simulink library "calc_radius_of_curvature"  (R2020a)
settings: Solver=VariableStepAuto  StartTime=0.0  StopTime=10.0  RelTol=1e-3
settings Model: Creator=Ayaz  LastModifiedBy=Ayaz

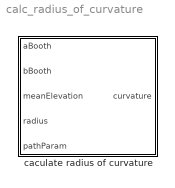
== system calc_radius_of_curvature ==
  caculate radius of curvature : Subsystem

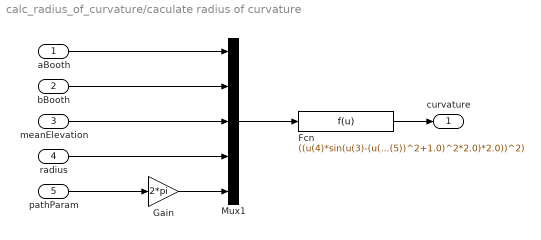
== system calc_radius_of_curvature/caculate radius of curvature ==
  aBooth : Inport
  bBooth : Inport  Port=2
  meanElevation : Inport  Port=3
  radius : Inport  Port=4
  pathParam : Inport  Port=5
  Fcn : Fcn  Expr=((u(4)*sin(u(3)-(u(1)^2*1.0/u(2)^2*cos(u(5))*sin(u(5)))/(u(1)^2*1.0/u(2)^2*cos(u(5))^2+1.0))*sin((u(1)*sin(u(5)))/(u(1)^2*1.0/u(2)^2*cos(u(5))^2+1.0))*((u(1)^2*1.0/u(2)^2*cos(u(5))^2)/(u(1)^2*1.0/u(2)^2*cos(u(5))^2+1.0)-(u(1)^2*1.0/u(2)^2*sin(u(5))^2)/(u(1)^2*1.0/u(2)^2*cos(u(5))^2+1.0)+u(1)^4*1.0/u(2)^4*cos(u(5))^2*sin(u(5))^2*1.0/(u(1)^2*1.0/u(2)^2*cos(u(5))^2+1.0)^2*2.0)+u(4)*cos(u(3)-(u(1)^2*1.0/u(2)^2*cos(u(5))*sin(u(5)))/(u(1)^2*1.0/u(2)^2*cos(u(5))^2+1.0))*cos((u(1)*sin(u(5)))/(u(1)^2*1.0/u(2)^2*cos(u(5))^2+1.0))*((u(1)*cos(u(5)))/(u(1)^2*1.0/u(2)^2*cos(u(5))^2+1.0)+u(1)^3*1.0/u(2)^2*cos(u(5))*sin(u(5))^2*1.0/(u(1)^2*1.0/u(2)^2*cos(u(5))^2+1.0)^2*2.0))^2+(u(4)*sin(u(3)-(u(1)^2*1.0/u(2)^2*cos(u(5))*sin(u(5)))/(u(1)^2*1.0/u(2)^2*cos(u(5))^2+1.0))*cos((u(1)*sin(u(5)))/(u(1)^2*1.0/u(2)^2*cos(u(5))^2+1.0))*((u(1)^2*1.0/u(2)^2*cos(u(5))^2)/(u(1)^2*1.0/u(2)^2*cos(u(5))^2+1.0)-(u(1)^2*1.0/u(2)^2*sin(u(5))^2)/(u(1)^2*1.0/u(2)^2*cos(u(5))^2+1.0)+u(1)^4*1.0/u(2)^4*cos(u(5))^2*sin(u(5))^2*1.0/(u(1)^2*1.0/u(2)^2*cos(u(5))^2+1.0)^2*2.0)-u(4)*cos(u(3)-(u(1)^2*1.0/u(2)^2*cos(u(5))*sin(u(5)))/(u(1)^2*1.0/u(2)^2*cos(u(5))^2+1.0))*sin((u(1)*sin(u(5)))/(u(1)^2*1.0/u(2)^2*cos(u(5))^2+1.0))*((u(1)*cos(u(5)))/(u(1)^2*1.0/u(2)^2*cos(u(5))^2+1.0)+u(1)^3*1.0/u(2)^2*cos(u(5))*sin(u(5))^2*1.0/(u(1)^2*1.0/u(2)^2*cos(u(5))^2+1.0)^2*2.0))^2+u(4)^2*cos(u(3)-(u(1)^2*1.0/u(2)^2*cos(u(5))*sin(u(5)))/(u(1)^2*1.0/u(2)^2*cos(u(5))^2+1.0))^2*((u(1)^2*1.0/u(2)^2*cos(u(5))^2)/(u(1)^2*1.0/u(2)^2*cos(u(5))^2+1.0)-(u(1)^2*1.0/u(2)^2*sin(u(5))^2)/(u(1)^2*1.0/u(2)^2*cos(u(5))^2+1.0)+u(1)^4*1.0/u(2)^4*cos(u(5))^2*sin(u(5))^2*1.0/(u(1)^2*1.0/u(2)^2*cos(u(5))^2+1.0)^2*2.0)^2)^(3.0/2.0)*1.0/sqrt(((u(4)*sin(u(3)-(u(1)^2*1.0/u(2)^2*cos(u(5))*sin(u(5)))/(u(1)^2*1.0/u(2)^2*cos(u(5))^2+1.0))*cos((u(1)*sin(u(5)))/(u(1)^2*1.0/u(2)^2*cos(u(5))^2+1.0))*((u(1)^2*1.0/u(2)^2*cos(u(5))^2)/(u(1)^2*1.0/u(2)^2*cos(u(5))^2+1.0)-(u(1)^2*1.0/u(2)^2*sin(u(5))^2)/(u(1)^2*1.0/u(2)^2*cos(u(5))^2+1.0)+u(1)^4*1.0/u(2)^4*cos(u(5))^2*sin(u(5))^2*1.0/(u(1)^2*1.0/u(2)^2*cos(u(5))^2+1.0)^2*2.0)-u(4)*cos(u(3)-(u(1)^2*1.0/u(2)^2*cos(u(5))*sin(u(5)))/(u(1)^2*1.0/u(2)^2*cos(u(5))^2+1.0))*sin((u(1)*sin(u(5)))/(u(1)^2*1.0/u(2)^2*cos(u(5))^2+1.0))*((u(1)*cos(u(5)))/(u(1)^2*1.0/u(2)^2*cos(u(5))^2+1.0)+u(1)^3*1.0/u(2)^2*cos(u(5))*sin(u(5))^2*1.0/(u(1)^2*1.0/u(2)^2*cos(u(5))^2+1.0)^2*2.0))*(u(4)*cos(u(3)-(u(1)^2*1.0/u(2)^2*cos(u(5))*sin(u(5)))/(u(1)^2*1.0/u(2)^2*cos(u(5))^2+1.0))*(u(1)^6*1.0/u(2)^6*cos(u(5))^3*sin(u(5))^3*1.0/(u(1)^2*1.0/u(2)^2*cos(u(5))^2+1.0)^3*8.0-(u(1)^2*1.0/u(2)^2*cos(u(5))*sin(u(5))*4.0)/(u(1)^2*1.0/u(2)^2*cos(u(5))^2+1.0)-u(1)^4*1.0/u(2)^4*cos(u(5))*sin(u(5))^3*1.0/(u(1)^2*1.0/u(2)^2*cos(u(5))^2+1.0)^2*6.0+u(1)^4*1.0/u(2)^4*cos(u(5))^3*sin(u(5))*1.0/(u(1)^2*1.0/u(2)^2*cos(u(5))^2+1.0)^2*6.0)+u(4)*sin(u(3)-(u(1)^2*1.0/u(2)^2*cos(u(5))*sin(u(5)))/(u(1)^2*1.0/u(2)^2*cos(u(5))^2+1.0))*((u(1)^2*1.0/u(2)^2*cos(u(5))^2)/(u(1)^2*1.0/u(2)^2*cos(u(5))^2+1.0)-(u(1)^2*1.0/u(2)^2*sin(u(5))^2)/(u(1)^2*1.0/u(2)^2*cos(u(5))^2+1.0)+u(1)^4*1.0/u(2)^4*cos(u(5))^2*sin(u(5))^2*1.0/(u(1)^2*1.0/u(2)^2*cos(u(5))^2+1.0)^2*2.0)^2)+u(4)*cos(u(3)-(u(1)^2*1.0/u(2)^2*cos(u(5))*sin(u(5)))/(u(1)^2*1.0/u(2)^2*cos(u(5))^2+1.0))*((u(1)^2*1.0/u(2)^2*cos(u(5))^2)/(u(1)^2*1.0/u(2)^2*cos(u(5))^2+1.0)-(u(1)^2*1.0/u(2)^2*sin(u(5))^2)/(u(1)^2*1.0/u(2)^2*cos(u(5))^2+1.0)+u(1)^4*1.0/u(2)^4*cos(u(5))^2*sin(u(5))^2*1.0/(u(1)^2*1.0/u(2)^2*cos(u(5))^2+1.0)^2*2.0)*(u(4)*cos(u(3)-(u(1)^2*1.0/u(2)^2*cos(u(5))*sin(u(5)))/(u(1)^2*1.0/u(2)^2*cos(u(5))^2+1.0))*cos((u(1)*sin(u(5)))/(u(1)^2*1.0/u(2)^2*cos(u(5))^2+1.0))*((u(1)^2*1.0/u(2)^2*cos(u(5))^2)/(u(1)^2*1.0/u(2)^2*cos(u(5))^2+1.0)-(u(1)^2*1.0/u(2)^2*sin(u(5))^2)/(u(1)^2*1.0/u(2)^2*cos(u(5))^2+1.0)+u(1)^4*1.0/u(2)^4*cos(u(5))^2*sin(u(5))^2*1.0/(u(1)^2*1.0/u(2)^2*cos(u(5))^2+1.0)^2*2.0)^2-u(4)*cos(u(3)-(u(1)^2*1.0/u(2)^2*cos(u(5))*sin(u(5)))/(u(1)^2*1.0/u(2)^2*cos(u(5))^2+1.0))*sin((u(1)*sin(u(5)))/(u(1)^2*1.0/u(2)^2*cos(u(5))^2+1.0))*((u(1)*sin(u(5)))/(u(1)^2*1.0/u(2)^2*cos(u(5))^2+1.0)+u(1)^3*1.0/u(2)^2*sin(u(5))^3*1.0/(u(1)^2*1.0/u(2)^2*cos(u(5))^2+1.0)^2*2.0-u(1)^5*1.0/u(2)^4*cos(u(5))^2*sin(u(5))^3*1.0/(u(1)^2*1.0/u(2)^2*cos(u(5))^2+1.0)^3*8.0-u(1)^3*1.0/u(2)^2*cos(u(5))^2*sin(u(5))*1.0/(u(1)^2*1.0/u(2)^2*cos(u(5))^2+1.0)^2*6.0)+u(4)*cos(u(3)-(u(1)^2*1.0/u(2)^2*cos(u(5))*sin(u(5)))/(u(1)^2*1.0/u(2)^2*cos(u(5))^2+1.0))*cos((u(1)*sin(u(5)))/(u(1)^2*1.0/u(2)^2*cos(u(5))^2+1.0))*((u(1)*cos(u(5)))/(u(1)^2*1.0/u(2)^2*cos(u(5))^2+1.0)+u(1)^3*1.0/u(2)^2*cos(u(5))*sin(u(5))^2*1.0/(u(1)^2*1.0/u(2)^2*cos(u(5))^2+1.0)^2*2.0)^2-u(4)*sin(u(3)-(u(1)^2*1.0/u(2)^2*cos(u(5))*sin(u(5)))/(u(1)^2*1.0/u(2)^2*cos(u(5))^2+1.0))*cos((u(1)*sin(u(5)))/(u(1)^2*1.0/u(2)^2*cos(u(5))^2+1.0))*(u(1)^6*1.0/u(2)^6*cos(u(5))^3*sin(u(5))^3*1.0/(u(1)^2*1.0/u(2)^2*cos(u(5))^2+1.0)^3*8.0-(u(1)^2*1.0/u(2)^2*cos(u(5))*sin(u(5))*4.0)/(u(1)^2*1.0/u(2)^2*cos(u(5))^2+1.0)-u(1)^4*1.0/u(2)^4*cos(u(5))*sin(u(5))^3*1.0/(u(1)^2*1.0/u(2)^2*cos(u(5))^2+1.0)^2*6.0+u(1)^4*1.0/u(2)^4*cos(u(5))^3*sin(u(5))*1.0/(u(1)^2*1.0/u(2)^2*cos(u(5))^2+1.0)^2*6.0)+u(4)*sin(u(3)-(u(1)^2*1.0/u(2)^2*cos(u(5))*sin(u(5)))/(u(1)^2*1.0/u(2)^2*cos(u(5))^2+1.0))*sin((u(1)*sin(u(5)))/(u(1)^2*1.0/u(2)^2*cos(u(5))^2+1.0))*((u(1)*cos(u(5)))/(u(1)^2*1.0/u(2)^2*cos(u(5))^2+1.0)+u(1)^3*1.0/u(2)^2*cos(u(5))*sin(u(5))^2*1.0/(u(1)^2*1.0/u(2)^2*cos(u(5))^2+1.0)^2*2.0)*((u(1)^2*1.0/u(2)^2*cos(u(5))^2)/(u(1)^2*1.0/u(2)^2*cos(u(5))^2+1.0)-(u(1)^2*1.0/u(2)^2*sin(u(5))^2)/(u(1)^2*1.0/u(2)^2*cos(u(5))^2+1.0)+u(1)^4*1.0/u(2)^4*cos(u(5))^2*sin(u(5))^2*1.0/(u(1)^2*1.0/u(2)^2*cos(u(5))^2+1.0)^2*2.0)*2.0))^2+((u(4)*sin(u(3)-(u(1)^2*1.0/u(2)^2*cos(u(5))*sin(u(5)))/(u(1)^2*1.0/u(2)^2*cos(u(5))^2+1.0))*sin((u(1)*sin(u(5)))/(u(1)^2*1.0/u(2)^2*cos(u(5))^2+1.0))*((u(1)^2*1.0/u(2)^2*cos(u(5))^2)/(u(1)^2*1.0/u(2)^2*cos(u(5))^2+1.0)-(u(1)^2*1.0/u(2)^2*sin(u(5))^2)/(u(1)^2*1.0/u(2)^2*cos(u(5))^2+1.0)+u(1)^4*1.0/u(2)^4*cos(u(5))^2*sin(u(5))^2*1.0/(u(1)^2*1.0/u(2)^2*cos(u(5))^2+1.0)^2*2.0)+u(4)*cos(u(3)-(u(1)^2*1.0/u(2)^2*cos(u(5))*sin(u(5)))/(u(1)^2*1.0/u(2)^2*cos(u(5))^2+1.0))*cos((u(1)*sin(u(5)))/(u(1)^2*1.0/u(2)^2*cos(u(5))^2+1.0))*((u(1)*cos(u(5)))/(u(1)^2*1.0/u(2)^2*cos(u(5))^2+1.0)+u(1)^3*1.0/u(2)^2*cos(u(5))*sin(u(5))^2*1.0/(u(1)^2*1.0/u(2)^2*cos(u(5))^2+1.0)^2*2.0))*(u(4)*cos(u(3)-(u(1)^2*1.0/u(2)^2*cos(u(5))*sin(u(5)))/(u(1)^2*1.0/u(2)^2*cos(u(5))^2+1.0))*(u(1)^6*1.0/u(2)^6*cos(u(5))^3*sin(u(5))^3*1.0/(u(1)^2*1.0/u(2)^2*cos(u(5))^2+1.0)^3*8.0-(u(1)^2*1.0/u(2)^2*cos(u(5))*sin(u(5))*4.0)/(u(1)^2*1.0/u(2)^2*cos(u(5))^2+1.0)-u(1)^4*1.0/u(2)^4*cos(u(5))*sin(u(5))^3*1.0/(u(1)^2*1.0/u(2)^2*cos(u(5))^2+1.0)^2*6.0+u(1)^4*1.0/u(2)^4*cos(u(5))^3*sin(u(5))*1.0/(u(1)^2*1.0/u(2)^2*cos(u(5))^2+1.0)^2*6.0)+u(4)*sin(u(3)-(u(1)^2*1.0/u(2)^2*cos(u(5))*sin(u(5)))/(u(1)^2*1.0/u(2)^2*cos(u(5))^2+1.0))*((u(1)^2*1.0/u(2)^2*cos(u(5))^2)/(u(1)^2*1.0/u(2)^2*cos(u(5))^2+1.0)-(u(1)^2*1.0/u(2)^2*sin(u(5))^2)/(u(1)^2*1.0/u(2)^2*cos(u(5))^2+1.0)+u(1)^4*1.0/u(2)^4*cos(u(5))^2*sin(u(5))^2*1.0/(u(1)^2*1.0/u(2)^2*cos(u(5))^2+1.0)^2*2.0)^2)+u(4)*cos(u(3)-(u(1)^2*1.0/u(2)^2*cos(u(5))*sin(u(5)))/(u(1)^2*1.0/u(2)^2*cos(u(5))^2+1.0))*((u(1)^2*1.0/u(2)^2*cos(u(5))^2)/(u(1)^2*1.0/u(2)^2*cos(u(5))^2+1.0)-(u(1)^2*1.0/u(2)^2*sin(u(5))^2)/(u(1)^2*1.0/u(2)^2*cos(u(5))^2+1.0)+u(1)^4*1.0/u(2)^4*cos(u(5))^2*sin(u(5))^2*1.0/(u(1)^2*1.0/u(2)^2*cos(u(5))^2+1.0)^2*2.0)*(-u(4)*sin(u(3)-(u(1)^2*1.0/u(2)^2*cos(u(5))*sin(u(5)))/(u(1)^2*1.0/u(2)^2*cos(u(5))^2+1.0))*sin((u(1)*sin(u(5)))/(u(1)^2*1.0/u(2)^2*cos(u(5))^2+1.0))*(u(1)^6*1.0/u(2)^6*cos(u(5))^3*sin(u(5))^3*1.0/(u(1)^2*1.0/u(2)^2*cos(u(5))^2+1.0)^3*8.0-(u(1)^2*1.0/u(2)^2*cos(u(5))*sin(u(5))*4.0)/(u(1)^2*1.0/u(2)^2*cos(u(5))^2+1.0)-u(1)^4*1.0/u(2)^4*cos(u(5))*sin(u(5))^3*1.0/(u(1)^2*1.0/u(2)^2*cos(u(5))^2+1.0)^2*6.0+u(1)^4*1.0/u(2)^4*cos(u(5))^3*sin(u(5))*1.0/(u(1)^2*1.0/u(2)^2*cos(u(5))^2+1.0)^2*6.0)+u(4)*cos(u(3)-(u(1)^2*1.0/u(2)^2*cos(u(5))*sin(u(5)))/(u(1)^2*1.0/u(2)^2*cos(u(5))^2+1.0))*cos((u(1)*sin(u(5)))/(u(1)^2*1.0/u(2)^2*cos(u(5))^2+1.0))*((u(1)*sin(u(5)))/(u(1)^2*1.0/u(2)^2*cos(u(5))^2+1.0)+u(1)^3*1.0/u(2)^2*sin(u(5))^3*1.0/(u(1)^2*1.0/u(2)^2*cos(u(5))^2+1.0)^2*2.0-u(1)^5*1.0/u(2)^4*cos(u(5))^2*sin(u(5))^3*1.0/(u(1)^2*1.0/u(2)^2*cos(u(5))^2+1.0)^3*8.0-u(1)^3*1.0/u(2)^2*cos(u(5))^2*sin(u(5))*1.0/(u(1)^2*1.0/u(2)^2*cos(u(5))^2+1.0)^2*6.0)+u(4)*cos(u(3)-(u(1)^2*1.0/u(2)^2*cos(u(5))*sin(u(5)))/(u(1)^2*1.0/u(2)^2*cos(u(5))^2+1.0))*sin((u(1)*sin(u(5)))/(u(1)^2*1.0/u(2)^2*cos(u(5))^2+1.0))*((u(1)^2*1.0/u(2)^2*cos(u(5))^2)/(u(1)^2*1.0/u(2)^2*cos(u(5))^2+1.0)-(u(1)^2*1.0/u(2)^2*sin(u(5))^2)/(u(1)^2*1.0/u(2)^2*cos(u(5))^2+1.0)+u(1)^4*1.0/u(2)^4*cos(u(5))^2*sin(u(5))^2*1.0/(u(1)^2*1.0/u(2)^2*cos(u(5))^2+1.0)^2*2.0)^2+u(4)*cos(u(3)-(u(1)^2*1.0/u(2)^2*cos(u(5))*sin(u(5)))/(u(1)^2*1.0/u(2)^2*cos(u(5))^2+1.0))*sin((u(1)*sin(u(5)))/(u(1)^2*1.0/u(2)^2*cos(u(5))^2+1.0))*((u(1)*cos(u(5)))/(u(1)^2*1.0/u(2)^2*cos(u(5))^2+1.0)+u(1)^3*1.0/u(2)^2*cos(u(5))*sin(u(5))^2*1.0/(u(1)^2*1.0/u(2)^2*cos(u(5))^2+1.0)^2*2.0)^2-u(4)*sin(u(3)-(u(1)^2*1.0/u(2)^2*cos(u(5))*sin(u(5)))/(u(1)^2*1.0/u(2)^2*cos(u(5))^2+1.0))*cos((u(1)*sin(u(5)))/(u(1)^2*1.0/u(2)^2*cos(u(5))^2+1.0))*((u(1)*cos(u(5)))/(u(1)^2*1.0/u(2)^2*cos(u(5))^2+1.0)+u(1)^3*1.0/u(2)^2*cos(u(5))*sin(u(5))^2*1.0/(u(1)^2*1.0/u(2)^2*cos(u(5))^2+1.0)^2*2.0)*((u(1)^2*1.0/u(2)^2*cos(u(5))^2)/(u(1)^2*1.0/u(2)^2*cos(u(5))^2+1.0)-(u(1)^2*1.0/u(2)^2*sin(u(5))^2)/(u(1)^2*1.0/u(2)^2*cos(u(5))^2+1.0)+u(1)^4*1.0/u(2)^4*cos(u(5))^2*sin(u(5))^2*1.0/(u(1)^2*1.0/u(2)^2*cos(u(5))^2+1.0)^2*2.0)*2.0))^2+((u(4)*sin(u(3)-(u(1)^2*1.0/u(2)^2*cos(u(5))*sin(u(5)))/(u(1)^2*1.0/u(2)^2*cos(u(5))^2+1.0))*sin((u(1)*sin(u(5)))/(u(1)^2*1.0/u(2)^2*cos(u(5))^2+1.0))*((u(1)^2*1.0/u(2)^2*cos(u(5))^2)/(u(1)^2*1.0/u(2)^2*cos(u(5))^2+1.0)-(u(1)^2*1.0/u(2)^2*sin(u(5))^2)/(u(1)^2*1.0/u(2)^2*cos(u(5))^2+1.0)+u(1)^4*1.0/u(2)^4*cos(u(5))^2*sin(u(5))^2*1.0/(u(1)^2*1.0/u(2)^2*cos(u(5))^2+1.0)^2*2.0)+u(4)*cos(u(3)-(u(1)^2*1.0/u(2)^2*cos(u(5))*sin(u(5)))/(u(1)^2*1.0/u(2)^2*cos(u(5))^2+1.0))*cos((u(1)*sin(u(5)))/(u(1)^2*1.0/u(2)^2*cos(u(5))^2+1.0))*((u(1)*cos(u(5)))/(u(1)^2*1.0/u(2)^2*cos(u(5))^2+1.0)+u(1)^3*1.0/u(2)^2*cos(u(5))*sin(u(5))^2*1.0/(u(1)^2*1.0/u(2)^2*cos(u(5))^2+1.0)^2*2.0))*(u(4)*cos(u(3)-(u(1)^2*1.0/u(2)^2*cos(u(5))*sin(u(5)))/(u(1)^2*1.0/u(2)^2*cos(u(5))^2+1.0))*cos((u(1)*sin(u(5)))/(u(1)^2*1.0/u(2)^2*cos(u(5))^2+1.0))*((u(1)^2*1.0/u(2)^2*cos(u(5))^2)/(u(1)^2*1.0/u(2)^2*cos(u(5))^2+1.0)-(u(1)^2*1.0/u(2)^2*sin(u(5))^2)/(u(1)^2*1.0/u(2)^2*cos(u(5))^2+1.0)+u(1)^4*1.0/u(2)^4*cos(u(5))^2*sin(u(5))^2*1.0/(u(1)^2*1.0/u(2)^2*cos(u(5))^2+1.0)^2*2.0)^2-u(4)*cos(u(3)-(u(1)^2*1.0/u(2)^2*cos(u(5))*sin(u(5)))/(u(1)^2*1.0/u(2)^2*cos(u(5))^2+1.0))*sin((u(1)*sin(u(5)))/(u(1)^2*1.0/u(2)^2*cos(u(5))^2+1.0))*((u(1)*sin(u(5)))/(u(1)^2*1.0/u(2)^2*cos(u(5))^2+1.0)+u(1)^3*1.0/u(2)^2*sin(u(5))^3*1.0/(u(1)^2*1.0/u(2)^2*cos(u(5))^2+1.0)^2*2.0-u(1)^5*1.0/u(2)^4*cos(u(5))^2*sin(u(5))^3*1.0/(u(1)^2*1.0/u(2)^2*cos(u(5))^2+1.0)^3*8.0-u(1)^3*1.0/u(2)^2*cos(u(5))^2*sin(u(5))*1.0/(u(1)^2*1.0/u(2)^2*cos(u(5))^2+1.0)^2*6.0)+u(4)*cos(u(3)-(u(1)^2*1.0/u(2)^2*cos(u(5))*sin(u(5)))/(u(1)^2*1.0/u(2)^2*cos(u(5))^2+1.0))*cos((u(1)*sin(u(5)))/(u(1)^2*1.0/u(2)^2*cos(u(5))^2+1.0))*((u(1)*cos(u(5)))/(u(1)^2*1.0/u(2)^2*cos(u(5))^2+1.0)+u(1)^3*1.0/u(2)^2*cos(u(5))*sin(u(5))^2*1.0/(u(1)^2*1.0/u(2)^2*cos(u(5))^2+1.0)^2*2.0)^2-u(4)*sin(u(3)-(u(1)^2*1.0/u(2)^2*cos(u(5))*sin(u(5)))/(u(1)^2*1.0/u(2)^2*cos(u(5))^2+1.0))*cos((u(1)*sin(u(5)))/(u(1)^2*1.0/u(2)^2*cos(u(5))^2+1.0))*(u(1)^6*1.0/u(2)^6*cos(u(5))^3*sin(u(5))^3*1.0/(u(1)^2*1.0/u(2)^2*cos(u(5))^2+1.0)^3*8.0-(u(1)^2*1.0/u(2)^2*cos(u(5))*sin(u(5))*4.0)/(u(1)^2*1.0/u(2)^2*cos(u(5))^2+1.0)-u(1)^4*1.0/u(2)^4*cos(u(5))*sin(u(5))^3*1.0/(u(1)^2*1.0/u(2)^2*cos(u(5))^2+1.0)^2*6.0+u(1)^4*1.0/u(2)^4*cos(u(5))^3*sin(u(5))*1.0/(u(1)^2*1.0/u(2)^2*cos(u(5))^2+1.0)^2*6.0)+u(4)*sin(u(3)-(u(1)^2*1.0/u(2)^2*cos(u(5))*sin(u(5)))/(u(1)^2*1.0/u(2)^2*cos(u(5))^2+1.0))*sin((u(1)*sin(u(5)))/(u(1)^2*1.0/u(2)^2*cos(u(5))^2+1.0))*((u(1)*cos(u(5)))/(u(1)^2*1.0/u(2)^2*cos(u(5))^2+1.0)+u(1)^3*1.0/u(2)^2*cos(u(5))*sin(u(5))^2*1.0/(u(1)^2*1.0/u(2)^2*cos(u(5))^2+1.0)^2*2.0)*((u(1)^2*1.0/u(2)^2*cos(u(5))^2)/(u(1)^2*1.0/u(2)^2*cos(u(5))^2+1.0)-(u(1)^2*1.0/u(2)^2*sin(u(5))^2)/(u(1)^2*1.0/u(2)^2*cos(u(5))^2+1.0)+u(1)^4*1.0/u(2)^4*cos(u(5))^2*sin(u(5))^2*1.0/(u(1)^2*1.0/u(2)^2*cos(u(5))^2+1.0)^2*2.0)*2.0)-(u(4)*sin(u(3)-(u(1)^2*1.0/u(2)^2*cos(u(5))*sin(u(5)))/(u(1)^2*1.0/u(2)^2*cos(u(5))^2+1.0))*cos((u(1)*sin(u(5)))/(u(1)^2*1.0/u(2)^2*cos(u(5))^2+1.0))*((u(1)^2*1.0/u(2)^2*cos(u(5))^2)/(u(1)^2*1.0/u(2)^2*cos(u(5))^2+1.0)-(u(1)^2*1.0/u(2)^2*sin(u(5))^2)/(u(1)^2*1.0/u(2)^2*cos(u(5))^2+1.0)+u(1)^4*1.0/u(2)^4*cos(u(5))^2*sin(u(5))^2*1.0/(u(1)^2*1.0/u(2)^2*cos(u(5))^2+1.0)^2*2.0)-u(4)*cos(u(3)-(u(1)^2*1.0/u(2)^2*cos(u(5))*sin(u(5)))/(u(1)^2*1.0/u(2)^2*cos(u(5))^2+1.0))*sin((u(1)*sin(u(5)))/(u(1)^2*1.0/u(2)^2*cos(u(5))^2+1.0))*((u(1)*cos(u(5)))/(u(1)^2*1.0/u(2)^2*cos(u(5))^2+1.0)+u(1)^3*1.0/u(2)^2*cos(u(5))*sin(u(5))^2*1.0/(u(1)^2*1.0/u(2)^2*cos(u(5))^2+1.0)^2*2.0))*(-u(4)*sin(u(3)-(u(1)^2*1.0/u(2)^2*cos(u(5))*sin(u(5)))/(u(1)^2*1.0/u(2)^2*cos(u(5))^2+1.0))*sin((u(1)*sin(u(5)))/(u(1)^2*1.0/u(2)^2*cos(u(5))^2+1.0))*(u(1)^6*1.0/u(2)^6*cos(u(5))^3*sin(u(5))^3*1.0/(u(1)^2*1.0/u(2)^2*cos(u(5))^2+1.0)^3*8.0-(u(1)^2*1.0/u(2)^2*cos(u(5))*sin(u(5))*4.0)/(u(1)^2*1.0/u(2)^2*cos(u(5))^2+1.0)-u(1)^4*1.0/u(2)^4*cos(u(5))*sin(u(5))^3*1.0/(u(1)^2*1.0/u(2)^2*cos(u(5))^2+1.0)^2*6.0+u(1)^4*1.0/u(2)^4*cos(u(5))^3*sin(u(5))*1.0/(u(1)^2*1.0/u(2)^2*cos(u(5))^2+1.0)^2*6.0)+u(4)*cos(u(3)-(u(1)^2*1.0/u(2)^2*cos(u(5))*sin(u(5)))/(u(1)^2*1.0/u(2)^2*cos(u(5))^2+1.0))*cos((u(1)*sin(u(5)))/(u(1)^2*1.0/u(2)^2*cos(u(5))^2+1.0))*((u(1)*sin(u(5)))/(u(1)^2*1.0/u(2)^2*cos(u(5))^2+1.0)+u(1)^3*1.0/u(2)^2*sin(u(5))^3*1.0/(u(1)^2*1.0/u(2)^2*cos(u(5))^2+1.0)^2*2.0-u(1)^5*1.0/u(2)^4*cos(u(5))^2*sin(u(5))^3*1.0/(u(1)^2*1.0/u(2)^2*cos(u(5))^2+1.0)^3*8.0-u(1)^3*1.0/u(2)^2*cos(u(5))^2*sin(u(5))*1.0/(u(1)^2*1.0/u(2)^2*cos(u(5))^2+1.0)^2*6.0)+u(4)*cos(u(3)-(u(1)^2*1.0/u(2)^2*cos(u(5))*sin(u(5)))/(u(1)^2*1.0/u(2)^2*cos(u(5))^2+1.0))*sin((u(1)*sin(u(5)))/(u(1)^2*1.0/u(2)^2*cos(u(5))^2+1.0))*((u(1)^2*1.0/u(2)^2*cos(u(5))^2)/(u(1)^2*1.0/u(2)^2*cos(u(5))^2+1.0)-(u(1)^2*1.0/u(2)^2*sin(u(5))^2)/(u(1)^2*1.0/u(2)^2*cos(u(5))^2+1.0)+u(1)^4*1.0/u(2)^4*cos(u(5))^2*sin(u(5))^2*1.0/(u(1)^2*1.0/u(2)^2*cos(u(5))^2+1.0)^2*2.0)^2+u(4)*cos(u(3)-(u(1)^2*1.0/u(2)^2*cos(u(5))*sin(u(5)))/(u(1)^2*1.0/u(2)^2*cos(u(5))^2+1.0))*sin((u(1)*sin(u(5)))/(u(1)^2*1.0/u(2)^2*cos(u(5))^2+1.0))*((u(1)*cos(u(5)))/(u(1)^2*1.0/u(2)^2*cos(u(5))^2+1.0)+u(1)^3*1.0/u(2)^2*cos(u(5))*sin(u(5))^2*1.0/(u(1)^2*1.0/u(2)^2*cos(u(5))^2+1.0)^2*2.0)^2-u(4)*sin(u(3)-(u(1)^2*1.0/u(2)^2*cos(u(5))*sin(u(5)))/(u(1)^2*1.0/u(2)^2*cos(u(5))^2+1.0))*cos((u(1)*sin(u(5)))/(u(1)^2*1.0/u(2)^2*cos(u(5))^2+1.0))*((u(1)*cos(u(5)))/(u(1)^2*1.0/u(2)^2*cos(u(5))^2+1.0)+u(1)^3*1.0/u(2)^2*cos(u(5))*sin(u(5))^2*1.0/(u(1)^2*1.0/u(2)^2*cos(u(5))^2+1.0)^2*2.0)*((u(1)^2*1.0/u(2)^2*cos(u(5))^2)/(u(1)^2*1.0/u(2)^2*cos(u(5))^2+1.0)-(u(1)^2*1.0/u(2)^2*sin(u(5))^2)/(u(1)^2*1.0/u(2)^2*cos(u(5))^2+1.0)+u(1)^4*1.0/u(2)^4*cos(u(5))^2*sin(u(5))^2*1.0/(u(1)^2*1.0/u(2)^2*cos(u(5))^2+1.0)^2*2.0)*2.0))^2)
  Gain : Gain  Gain=2*pi
  Mux1 : Mux  Inputs=5
  curvature : Outport
  wires:
  aBooth/1 -> Mux1/1
  radius/1 -> Mux1/4
  Mux1/1 -> Fcn/1
  Fcn/1 -> curvature/1
  bBooth/1 -> Mux1/2
  meanElevation/1 -> Mux1/3
  Gain/1 -> Mux1/5
  pathParam/1 -> Gain/1
